simulink model "trajectoryGeneration"  (R2021b)
settings: Solver=ode1  StartTime=0.0  StopTime=10.0  RelTol=1e-3
settings Model: Creator=ATLabor  LastModifiedBy=ATLabor
settings OptimizationCC: DefaultParameterBehavior=Inlined  LocalBlockOutputs=off
settings RTWCC: Description=TwinCAT GRT Target  SystemTargetFile=TwinCatGrt.tlc  TemplateMakefile=tcgrt_msbuild.tmf  TargetLang=C++
settings STFCustomTargetCC: TargetLangStandard=C++11 (ISO)  CombineOutputUpdateFcns=on  CodeInterfacePackaging=Reusable function  CPPClassGenCompliant=on  GRTInterface=off  GenerateAllocFcn=on  SystemTargetFile=TwinCatGrt.tlc
settings GRTTargetCC: TargetLangStandard=C++11 (ISO)  ParMdlRefBuildCompliant=off  CompOptLevelCompliant=off  ConcurrentExecutionCompliant=off  MatFileLogging=off  CodeInterfacePackaging=Reusable function  GenerateAllocFcn=on  UseToolchainInfoCompliant=off  ExtModeMexFile=TcExtModeClient

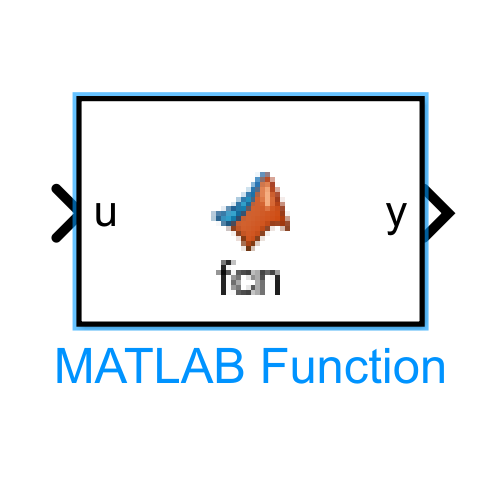
[thumbnail: Simulink's stored preview of the top-level diagram]
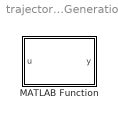
== system trajectoryGeneration ==
  MATLAB Function : MATLAB Function  TreatAsAtomicUnit=on

== matlab function trajectoryGeneration/MATLAB Function ==
  data: u input; y output
function y = fcn(u)
    u = 1;
    y = [1000,1000,1000,1500,2000,2000,2000,1500,1000]/1000;
    x = [1000,3000,5000,5000,5000,3000,1000,1000,1000]/1000;
    path = Path(x,y,0.4);
y = u;
